simulink model "motor"  (R2020a)
settings: Solver=VariableStepAuto  StartTime=0.0  StopTime=10.0  RelTol=1e-3
undefined symbols (not defined in the file): Rr, Rs
settings Model: Creator=Laza  LastModifiedBy=Laza

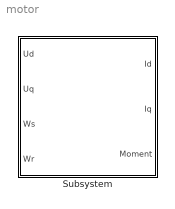
== system motor ==
  Subsystem : Subsystem

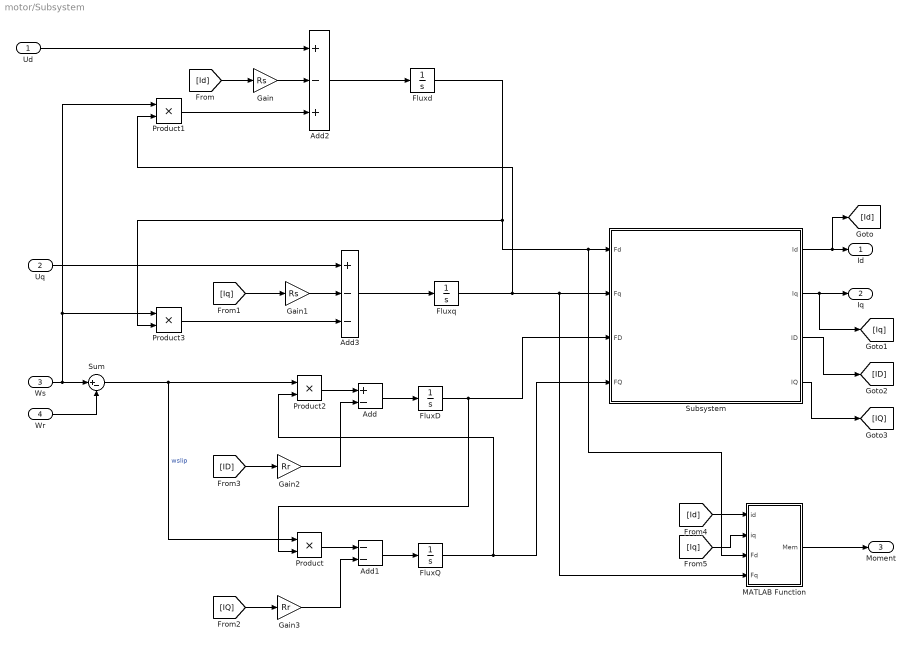
== system motor/Subsystem ==
  Ud : Inport
  Uq : Inport  Port=2
  Ws : Inport  Port=3
  Wr : Inport  Port=4
  Add : Sum  Inputs=+-
  Add1 : Sum  Inputs=--
  Add2 : Sum  Inputs=+-+
  Add3 : Sum  Inputs=+--
  FluxD : Integrator
  FluxQ : Integrator
  Fluxd : Integrator
  Fluxq : Integrator
  Gain : Gain  Gain=Rs
  Gain1 : Gain  Gain=Rs
  Gain2 : Gain  Gain=Rr
  Gain3 : Gain  Gain=Rr
  MATLAB Function : MATLAB Function  TreatAsAtomicUnit=on
  Product{,1..3} (4 alike) : Product
  Subsystem : Subsystem
  Sum : Sum  Inputs=|+-
  Id : Outport
  Iq : Outport  Port=2
  Moment : Outport  Port=3
  wires:
  Uq/1 -> Add3/1
  Wr/1 -> Sum/2
  Add/1 -> FluxD/1
  Add1/1 -> FluxQ/1
  Product/1 -> Add1/1
  Gain3/1 -> Add1/2
  Product2/1 -> Add/1
  Gain2/1 -> Add/2
  Sum/1 -> Product/1, Product2/1  "wslip"
  Add2/1 -> Fluxd/1
  Add3/1 -> Fluxq/1
  Ud/1 -> Add2/1
  Fluxd/1 -> Product3/2, MATLAB Function/3(Fd), Subsystem/1(Fd)
  Fluxq/1 -> Product1/2, MATLAB Function/4(Fq), Subsystem/2(Fq)
  FluxD/1 -> Product/2, Subsystem/3(FD)
  FluxQ/1 -> Product2/2, Subsystem/4(FQ)
  Subsystem/2(Iq) -> [Iq], Iq/1
  Gain/1 -> Add2/2
  Subsystem/1(Id) -> [Id], Id/1
  Gain1/1 -> Add3/2
  [Id] -> Gain/1
  [Iq] -> Gain1/1
  Subsystem/3(ID) -> [ID]
  Subsystem/4(IQ) -> [IQ]
  [IQ] -> Gain3/1
  [ID] -> Gain2/1
  Product1/1 -> Add2/3
  Product3/1 -> Add3/3
  Ws/1 -> Product1/1, Product3/1, Sum/1
  MATLAB Function/1(Mem) -> Moment/1
  [Id] -> MATLAB Function/1(id)
  [Iq] -> MATLAB Function/2(iq)

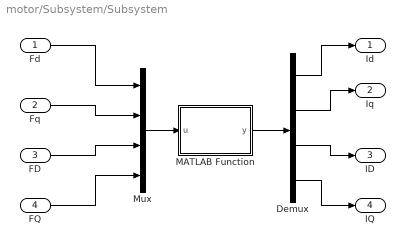
== system motor/Subsystem/Subsystem ==
  Fd : Inport
  Fq : Inport  Port=2
  FD : Inport  Port=3
  FQ : Inport  Port=4
  Demux : Demux
  MATLAB Function : MATLAB Function  TreatAsAtomicUnit=on
  Mux : Mux
  Id : Outport
  Iq : Outport  Port=2
  ID : Outport  Port=3
  IQ : Outport  Port=4
  wires:
  Demux/4 -> IQ/1
  Demux/3 -> ID/1
  Demux/2 -> Iq/1
  Demux/1 -> Id/1
  MATLAB Function/1(y) -> Demux/1
  Mux/1 -> MATLAB Function/1(u)
  Fd/1 -> Mux/1
  Fq/1 -> Mux/2
  FD/1 -> Mux/3
  FQ/1 -> Mux/4

== matlab function motor/Subsystem/MATLAB Function ==
  data: id input; Mem output; iq input; Fd input; Fq input
function Mem = fcn(id,iq,Fd,Fq)

Mem = 3/2*(Fd*iq-Fq*id);

== matlab function motor/Subsystem/Subsystem/MATLAB Function ==
  data: u input; y output
function y = fcn(u)
Ls=0.002;
Lr=0.001;
Lm=1e-5;
A=[Ls 0 Lm 0;...
   0 Ls 0 Lm;...
   Lm 0 Lr 0;...
   0 Lm 0 Lr]
y = inv(A)*u;
